simulink model "Delta_Sigma_ADC_Deg1"  (R2025b)
settings: Solver=VariableStepAuto  StartTime=0.0  StopTime=25  RelTol=1e-3
undefined symbols (not defined in the file): CURRENT_OSR, DiscIntNeverNeededParam
settings Model: Creator=Yash  LastModifiedBy=Yash

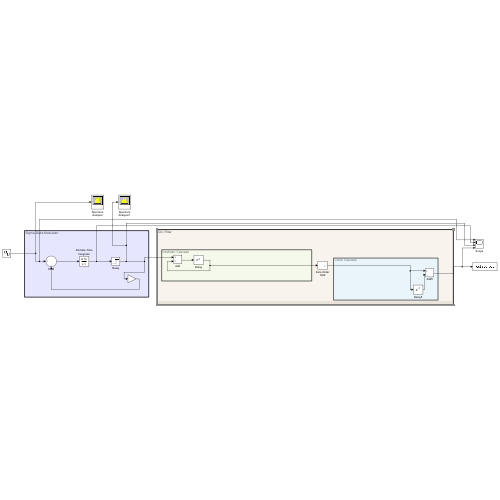
[thumbnail: Simulink's stored preview of the top-level diagram]
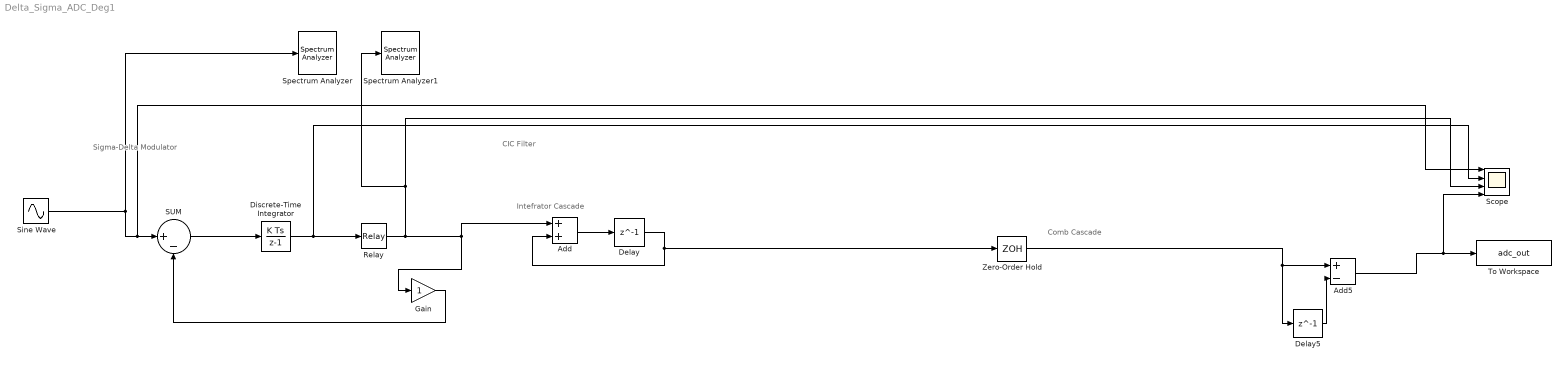
== system Delta_Sigma_ADC_Deg1 ==
  note: Sigma-Delta Modulator
  note: Intefrator Cascade
  note: CIC Filter
  note: Comb Cascade
  Add : Sum
  Add5 : Sum  Inputs=+-
  Delay : Delay  DelayLength=1
  Delay5 : Delay  DelayLength=1
  Discrete-Time Integrator : DiscreteIntegrator  SampleTime=1/128000  ICPrevOutput=DiscIntNeverNeededParam  ICPrevScaledInput=DiscIntNeverNeededParam
  Gain : Gain
  Relay : Relay  OnSwitchValue=0  OffSwitchValue=0  OffOutputValue=-1
  SUM : Sum  Inputs=|+-
  Scope : Scope  NumInputPorts=4
      settings: ActiveDisplayYMinimum=-0.87499999999381883  ActiveDisplayYMaximum=0.87499999999757749
  Sine Wave : Sin  Amplitude=0.7  SampleTime=1/128000
  Spectrum Analyzer : SpectrumAnalyzer  WindowPosition=[385.000000,40.000000,766.000000,785.000000,]  ScopeFrameLocation=window  Method=Welch  PlotAsTwoSidedSpectrum=off  FrequencyScale=Log  AveragingMethod=Exponential  YLimits=[-347.1939 57.8558]  SelectedToolstripTab=spectrumAnalyzerToolstrip.spectrumTab
  Spectrum Analyzer1 : SpectrumAnalyzer  WindowPosition=[385.000000,40.000000,766.000000,785.000000,]  ScopeFrameLocation=window  Method=Welch  PlotAsTwoSidedSpectrum=off  FrequencyScale=Log  AveragingMethod=Exponential  YLimits=[-62.0926 26.1777]  SelectedToolstripTab=spectrumAnalyzerToolstrip.spectrumTab
  To Workspace : ToWorkspace  VariableName=adc_out  SampleTime=-1
  Zero-Order Hold : ZeroOrderHold  SampleTime=CURRENT_OSR/128000
  wires:
  Relay/1 -> Gain/1, Add/1, Spectrum Analyzer1/1, Scope/3
  Add/1 -> Delay/1
  Gain/1 -> SUM/2
  Zero-Order Hold/1 -> Delay5/1, Add5/1
  Sine Wave/1 -> Scope/1, SUM/1, Spectrum Analyzer/1
  Discrete-Time Integrator/1 -> Scope/2, Relay/1
  Delay5/1 -> Add5/2
  SUM/1 -> Discrete-Time Integrator/1
  Delay/1 -> Zero-Order Hold/1, Add/2
  Add5/1 -> Scope/4, To Workspace/1
